simulink model "compliance_control"  (R2020b)
settings: Solver=VariableStepAuto  StartTime=0.0  StopTime=10  RelTol=1e-3
undefined symbols (not defined in the file): dqi, g_q, K, KD, KP, myRobot, qi, Ts, xd, xr
libraries: vrlib x1
settings Model: Creator=simon  LastModifiedBy=SimoneCremasco

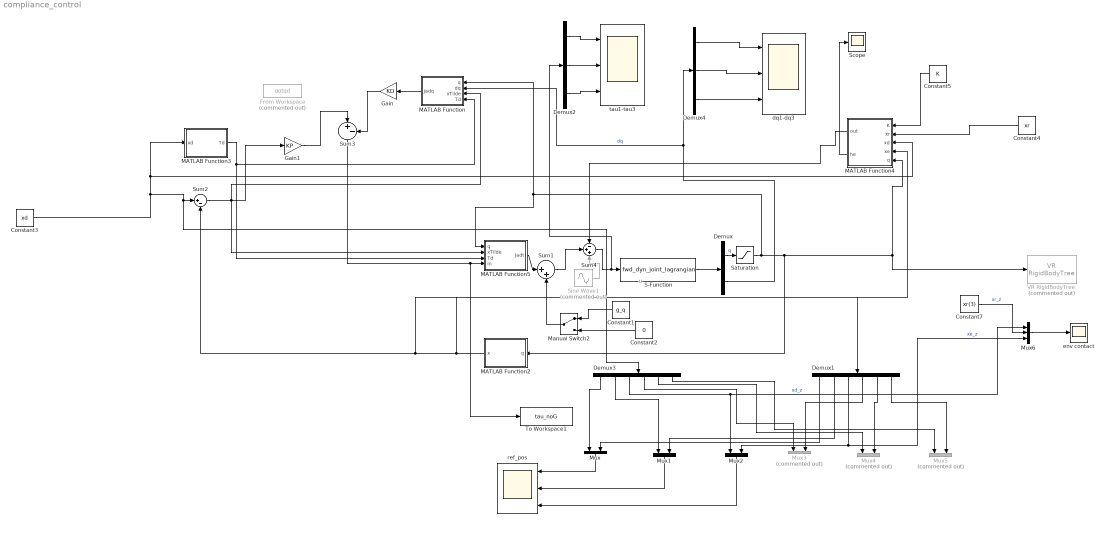
== system compliance_control ==
  note: u
  Constant1 : Constant  Value=g_q
  Constant2 : Constant  Value=0
  Constant3 : Constant  Value=xd
  Constant4 : Constant  Value=xr
  Constant5 : Constant  Value=K
  Constant7 : Constant  Value=xr(3)
  Demux : Demux  Outputs=2
  Demux1 : Demux  Outputs=6
  Demux2 : Demux  Outputs=myRobot.N
  Demux3 : Demux  Outputs=6
  Demux4 : Demux  Outputs=myRobot.N
  From Workspace : FromWorkspace  Commented=on  VariableName=dotqd  SampleTime=Ts
  Gain : Gain  Gain=KD
  Gain1 : Gain  Gain=KP
  MATLAB Function : MATLAB Function  TreatAsAtomicUnit=on
  MATLAB Function2 : MATLAB Function  TreatAsAtomicUnit=on
  MATLAB Function3 : MATLAB Function  TreatAsAtomicUnit=on
  MATLAB Function4 : MATLAB Function  TreatAsAtomicUnit=on
  MATLAB Function5 : MATLAB Function  TreatAsAtomicUnit=on
  Manual Switch2 : ManualSwitch
  Mux : Mux  Inputs=2
  Mux1 : Mux  Inputs=2
  Mux2 : Mux  Inputs=2
  Mux3 : Mux  Commented=on  Inputs=2
  Mux4 : Mux  Commented=on  Inputs=2
  Mux5 : Mux  Commented=on  Inputs=2
  Mux6 : Mux  Inputs=3
  S-Function : S-Function  FunctionName=fwd_dyn_joint_lagrangian  Parameters=myRobot,qi,dqi  SFunctionDeploymentMode=off  EnableBusSupport=off
  Saturation : Saturate  UpperLimit=[0.35 pi/2 0.2]  LowerLimit=[-0.35 -pi/2 -0.2]
  Scope : Scope
  Sine Wave1 : Sin  Commented=on  Amplitude=0.1  Frequency=5  SampleTime=0
  Sum1 : Sum  Inputs=|++
  Sum2 : Sum  Inputs=|+-
  Sum3 : Sum  Inputs=|+-
  Sum4 : Sum  Inputs=-++
  To Workspace1 : ToWorkspace  VariableName=tau_noG  SaveFormat=Timeseries  SampleTime=-1
  VR RigidBodyTree : vrlib/VR RigidBodyTree  Commented=on  RBT=rbt  useRBT=on  Ts=-1  ForceViewerOpen=on
      settings: SourceProductBaseCode=SL
  dq1-dq3 : Scope  NumInputPorts=3
  env contact : Scope
  ref_pos : Scope  NumInputPorts=3
  tau1-tau3 : Scope  NumInputPorts=3
  wires:
  Constant1/1 -> Manual Switch2/1
  Constant2/1 -> Manual Switch2/2
  Mux2/1 -> ref_pos/3
  Demux3/2 -> Mux1/1
  Mux1/1 -> ref_pos/2
  Demux3/1 -> Mux/1
  Mux/1 -> ref_pos/1
  Sum4/1 -> Demux2/1, S-Function/1
  Demux2/3 -> tau1-tau3/3
  Constant3/1 -> Demux3/1, Sum2/1, MATLAB Function3/1(xd), MATLAB Function4/3(xd)
  Manual Switch2/1 -> Sum1/2
  Sum1/1 -> Sum4/2
  Demux1/3 -> Mux2/2, Mux6/3  "xe_z"
  Demux4/1 -> dq1-dq3/1
  Demux4/3 -> dq1-dq3/3
  Demux/1 -> Saturation/1  "q"
  Sum2/1 -> MATLAB Function/3(xTilde), MATLAB Function5/2(xTilde), Gain1/1
  Demux4/2 -> dq1-dq3/2
  Gain1/1 -> Sum3/1
  Demux1/1 -> Mux/2
  Sum3/1 -> To Workspace1/1, MATLAB Function5/4(in)
  Demux3/3 -> Mux6/1, Mux2/1  "xd_z"
  S-Function/1 -> Demux/1
  Demux/2 -> MATLAB Function/2(dq), Demux4/1  "dq"
  Gain/1 -> Sum3/2
  Demux1/2 -> Mux1/2
  Demux2/1 -> tau1-tau3/1
  Demux2/2 -> tau1-tau3/2
  MATLAB Function/1(Jadq) -> Gain/1
  MATLAB Function5/1(Jadt) -> Sum1/1
  MATLAB Function2/1(x) -> MATLAB Function4/4(xe), Sum2/2, Demux1/1
  Demux1/5 -> Mux4/2
  Demux3/4 -> Mux3/1
  Demux3/5 -> Mux4/1
  Demux1/6 -> Mux5/2
  Demux1/4 -> Mux3/2
  Demux3/6 -> Mux5/1
  MATLAB Function3/1(Td) -> MATLAB Function/4(Td), MATLAB Function5/3(Td)
  Sine Wave1/1 -> Sum4/3
  MATLAB Function4/1(out) -> Sum4/1
  Constant4/1 -> MATLAB Function4/2(xr)
  Constant5/1 -> MATLAB Function4/1(K)
  Mux6/1 -> env contact/1
  Constant7/1 -> Mux6/2  "xr_z"
  MATLAB Function4/2(he) -> Scope/1
  Saturation/1 -> MATLAB Function/1(q), MATLAB Function5/1(q), VR RigidBodyTree/1, MATLAB Function4/5(q), MATLAB Function2/1(q)

== matlab function compliance_control/MATLAB Function ==
  data: q input size=3; Jadq output size=6; dq input; xTilde input; Td input
function Jadq = fcn(q, dq,xTilde, Td)

Jadq =getJad(q,xTilde,Td)*dq;

== matlab function compliance_control/MATLAB Function2 ==
  data: q input; x output
function x = fcn(q)
x = getK(q);

== matlab function compliance_control/MATLAB Function3 ==
  data: xd input; Td output
function Td = getTd(xd)
Rd = eul2rotm(xd(4:6)','ZYZ');
t = xd(1:3);
Td = [Rd t
    zeros(1,3) 1];

== matlab function compliance_control/MATLAB Function4 ==
  data: K input; out output size=3; xr input; xd input; xe input; q input; he output
function [out, he]= he(K, xr, xd, xe, q)
%consider the interaction only in z direction
if xe(3) < xr(3)
    dxrd = xd-xr;
    dxed = xd-xe;
    dxre = dxrd-dxed;
    he = K*dxre;
else
    he = zeros(6,1);
end
q2 = q(2);
Jtransp = [
[           0,         1.0,   0, 0, 0,   0]
[-0.3*sin(q2), 0.3*cos(q2),   0, 0, 0, 1.0]
[           0,           0, 1.0, 0, 0,   0]    
];
out = Jtransp*he;

== matlab function compliance_control/MATLAB Function5 ==
  data: q input size=3; Jadt output size=3; xTilde input; Td input; in input
function Jadt = fcn(q, xTilde, Td, in)

Jadt =getJad(q,xTilde,Td)'*in;
